simulink model "open_loop_experiments_R2018b"  (R2018b)
settings: Solver=ode45  StartTime=0.0  StopTime=simulation_time  MaxStep=0.01  RelTol=1e-3  EnableMultiTasking=on
values from neighbouring files (symbols this model uses):
  A = zeros(5,5)    [ex1.m]
  B = zeros(5,2)    [ex1.m]
  C = eye(5)    [ex1.m]    (also in exercise2_LQRandObserver.m = Corig)
  D = zeros(5,2)    [ex1.m]
  parameters = sol.getSystemParameters    [exercise1_Linearization.m]    (also in exercise2_LQRandObserver.m = sol1.getSystemParameters)
  path_to_track = ut.genCircularPath(curvature)    [exercise1_Linearization.m]
  Phi = eye(5) + A.*sampling_time*Psi    [ex1.m]
  sampling_time = 0.1    [exercise1_Linearization.m]    (also in exercise2_LQRandObserver.m = 0.01)
  x0 = {x0_experiment_1}    [ex1.m]    (also in exercise1_Linearization.m = x0_experiments{exp_id})
  x0_tild = x0Tild_experiments{exp_id}    [exercise1_Linearization.m]
undefined symbols (not defined in the file or in its folder): Gam
settings Model: Creator=ezequiel  LastModifiedBy=jianh
settings OptimizationCC: LifeSpan=inf
settings DebuggingCC: AllowSymbolicDim=off  SFUnexpectedBacktrackingDiag=warning  SFNoUnconditionalDefaultTransitionDiag=warning  SFExecutionAtInitializationDiag=none
settings ModelReferenceCC: PropagateSignalLabelsOutOfModel=off
settings SFSimCC: SimUseLocalCustomCode=off
settings RTWCC: RTWUseLocalCustomCode=off
settings CodeAppCC: StateflowObjectComments=on
settings GRTTargetCC: TargetLangStandard=C89/C90 (ANSI)
settings ConfigComp: CovMetricSettings=dw  CovHtmlReporting=on  CovSaveCumulativeToWorkspaceVar=on  CovSaveSingleToWorkspaceVar=on  CovExternalEMLEnable=off

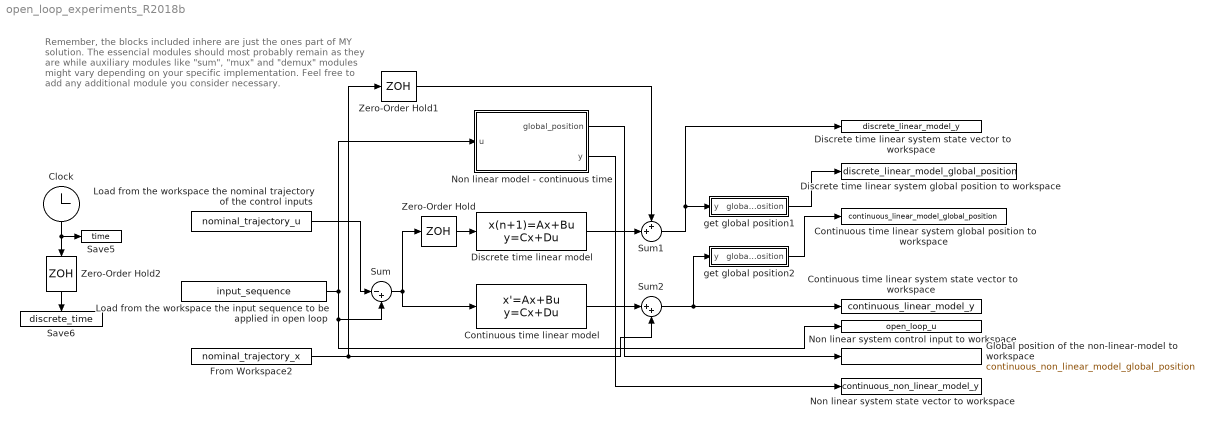
== system open_loop_experiments_R2018b ==
  note: Remember, the blocks included inhere are just the ones part of MY solution. The essencial modules should most probably remain as they are while auxiliary modules like "sum", "mux" and "demux" modules might vary depending on your specific implementation.
      |
      | Feel free to add any additional module you consider necessary.
  " Discrete time linear system state vector to workspace" : ToWorkspace  VariableName=discrete_linear_model_y  SampleTime=-1
  Clock : Clock
  Continuous time linear model : StateSpace  A=A  B=B  C=C  D=D  InitialCondition=x0_tild
  Continuous time linear system global position to workspace : ToWorkspace  VariableName=continuous_linear_model_global_position  SampleTime=-1
  Continuous time linear system state vector to workspace : ToWorkspace  VariableName=continuous_linear_model_y  SampleTime=-1
  Discrete time linear model : DiscreteStateSpace  A=Phi  B=Gam  C=C  D=D  InitialCondition=x0_tild  SampleTime=sampling_time
  Discrete time linear system global position to workspace : ToWorkspace  VariableName=discrete_linear_model_global_position  SampleTime=-1
  From Workspace2 : FromWorkspace  VariableName=nominal_trajectory_x  SampleTime=sampling_time  Interpolate=off  OutputAfterFinalValue=Holding final value
  Global position of the non-linear-model to workspace : ToWorkspace  VariableName=continuous_non_linear_model_global_position  SampleTime=-1
  Load from the workspace the input sequence to be applied in open loop : FromWorkspace  VariableName=input_sequence  SampleTime=sampling_time
  Load from the workspace the nominal trajectory of the control inputs : FromWorkspace  VariableName=nominal_trajectory_u  SampleTime=sampling_time  Interpolate=off  OutputAfterFinalValue=Holding final value
  Non linear model - continuous time : Subsystem
  Non linear system control input to workspace : ToWorkspace  VariableName=open_loop_u  SampleTime=-1
  Non linear system state vector to workspace : ToWorkspace  VariableName=continuous_non_linear_model_y  SampleTime=-1
  Save5 : ToWorkspace  VariableName=time  SampleTime=-1
  Save6 : ToWorkspace  VariableName=discrete_time  SampleTime=-1
  Sum : Sum  Inputs=|-+
  Sum1 : Sum  Inputs=++|
  Sum2 : Sum  Inputs=|++
  Zero-Order Hold : ZeroOrderHold  SampleTime=sampling_time
  Zero-Order Hold1 : ZeroOrderHold  SampleTime=sampling_time
  Zero-Order Hold2 : ZeroOrderHold  SampleTime=sampling_time
  get global position1 : Subsystem
  get global position2 : Subsystem
  wires:
  Clock/1 -> Save5/1, Zero-Order Hold2/1
  Zero-Order Hold2/1 -> Save6/1
  Non linear model - continuous time/1(global_position) -> Global position of the non-linear-model to workspace/1
  Sum/1 -> Continuous time linear model/1, Zero-Order Hold/1
  Zero-Order Hold/1 -> Discrete time linear model/1
  get global position1/1(global_position) -> Discrete time linear system global position to workspace/1
  get global position2/1(global_position) -> Continuous time linear system global position to workspace/1
  Non linear model - continuous time/2(y) -> Non linear system state vector to workspace/1
  Load from the workspace the nominal trajectory of the control inputs/1 -> Sum/1
  Load from the workspace the input sequence to be applied in open loop/1 -> Non linear model - continuous time/1(u), Non linear system control input to workspace/1, Sum/2
  Discrete time linear model/1 -> Sum1/2
  Sum1/1 -> " Discrete time linear system state vector to workspace"/1, get global position1/1(y)
  Continuous time linear model/1 -> Sum2/1
  Sum2/1 -> Continuous time linear system state vector to workspace/1, get global position2/1(y)
  From Workspace2/1 -> Zero-Order Hold1/1, Sum2/2
  Zero-Order Hold1/1 -> Sum1/1

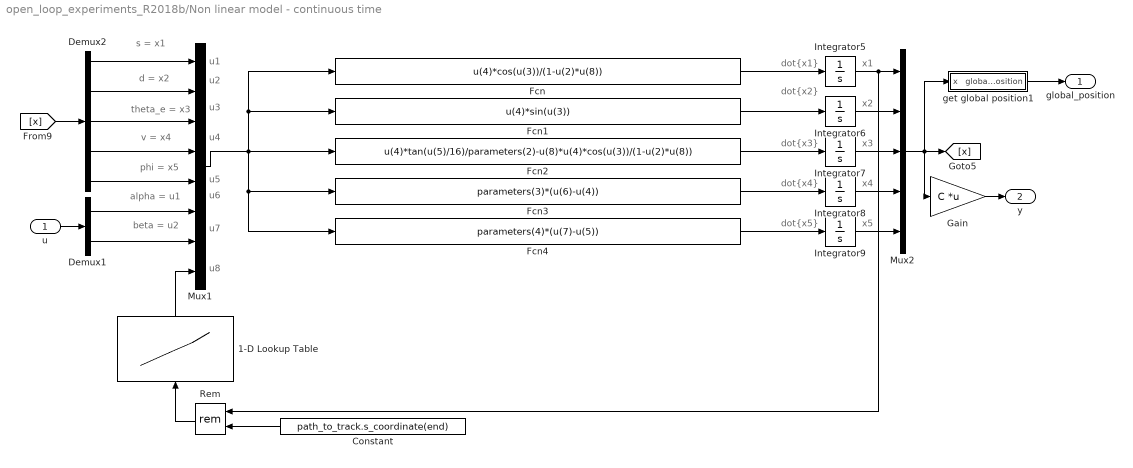
== system open_loop_experiments_R2018b/Non linear model - continuous time ==
  note: s = x1
  note: dot{x1}
  note: d = x2
  note: theta_e = x3
  note: v = x4
  note: phi = x5
  note: alpha = u1
  note: beta = u2
  note: u1
  note: u2
  note: u3
  note: u4
  note: u5
  note: u6
  note: u7
  note: x1
  note: dot{x2}
  note: x2
  note: dot{x3}
  note: x3
  note: dot{x4}
  note: x4
  note: dot{x5}
  note: x5
  note: u8
  u : Inport
  1-D Lookup Table : Lookup_n-D  NumberOfTableDimensions=1  BreakpointsForDimension1=path_to_track.s_coordinate  Table=path_to_track.curvature  InternalRulePriority=Speed  RndMeth=Simplest  InputSameDT=on
  Constant : Constant  Value=path_to_track.s_coordinate(end)
  Demux1 : Demux  Outputs=2
  Demux2 : Demux  Outputs=5
  Fcn : Fcn  Expr=u(4)*cos(u(3))/(1-u(2)*u(8))
  Fcn1 : Fcn  Expr=u(4)*sin(u(3))
  Fcn2 : Fcn  Expr=u(4)*tan(u(5)/16)/parameters(2)-u(8)*u(4)*cos(u(3))/(1-u(2)*u(8))
  Fcn3 : Fcn  Expr=parameters(3)*(u(6)-u(4))
  Fcn4 : Fcn  Expr=parameters(4)*(u(7)-u(5))
  Gain : Gain  Gain=C  Multiplication=Matrix(K*u)
  Integrator5 : Integrator  InitialCondition=x0(1)
  Integrator6 : Integrator  InitialCondition=x0(2)
  Integrator7 : Integrator  InitialCondition=x0(3)
  Integrator8 : Integrator  InitialCondition=x0(4)
  Integrator9 : Integrator  InitialCondition=x0(5)
  Mux1 : Mux  Inputs=8
  Mux2 : Mux  Inputs=5
  Rem : Math  Operator=rem  SaturateOnIntegerOverflow=on
  get global position1 : Subsystem
  global_position : Outport
  y : Outport  Port=2
  wires:
  u/1 -> Demux1/1
  Fcn/1 -> Integrator5/1
  Demux2/1 -> Mux1/1
  Demux2/2 -> Mux1/2
  Demux2/3 -> Mux1/3
  Demux2/4 -> Mux1/4
  Demux2/5 -> Mux1/5
  Demux1/1 -> Mux1/6
  Demux1/2 -> Mux1/7
  Mux1/1 -> Fcn3/1, Fcn4/1, Fcn1/1, Fcn/1, Fcn2/1
  Fcn1/1 -> Integrator6/1
  Integrator6/1 -> Mux2/2
  Fcn2/1 -> Integrator7/1
  Integrator7/1 -> Mux2/3
  Fcn3/1 -> Integrator8/1
  Integrator8/1 -> Mux2/4
  Fcn4/1 -> Integrator9/1
  Integrator9/1 -> Mux2/5
  [x] -> Demux2/1
  1-D Lookup Table/1 -> Mux1/8
  Rem/1 -> 1-D Lookup Table/1
  Constant/1 -> Rem/2
  Integrator5/1 -> Rem/1, Mux2/1
  Mux2/1 -> Gain/1, get global position1/1(x), [x]
  get global position1/1(global_position) -> global_position/1
  Gain/1 -> y/1

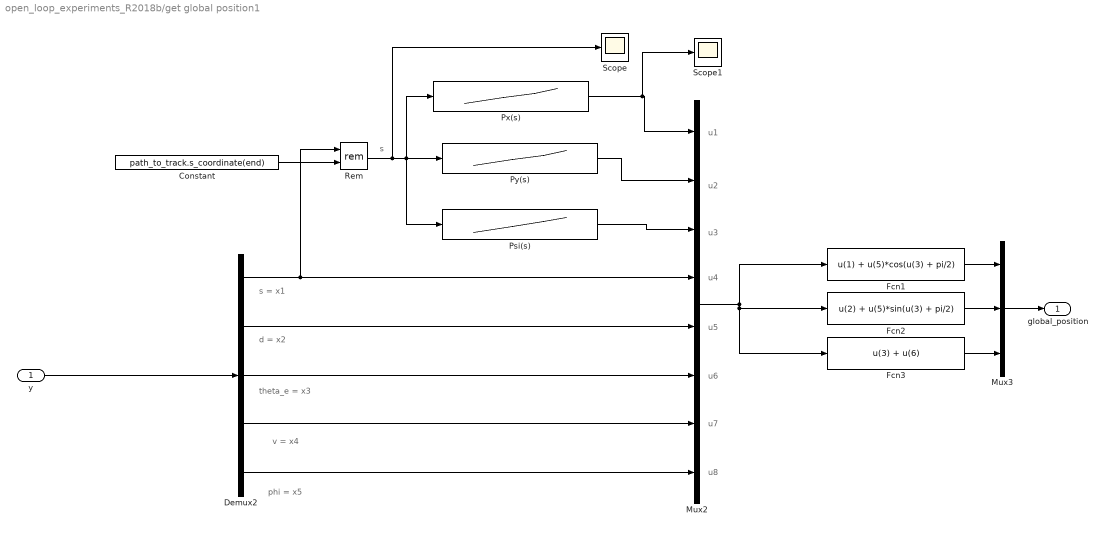
== system open_loop_experiments_R2018b/get global position1 ==
  note: s
  note: s = x1
  note: d = x2
  note: theta_e = x3
  note: v = x4
  note: phi = x5
  note: u1
  note: u2
  note: u3
  note: u4
  note: u5
  note: u6
  note: u7
  note: u8
  y : Inport
  Constant : Constant  Value=path_to_track.s_coordinate(end)
  Demux2 : Demux  Outputs=5
  Fcn1 : Fcn  Expr=u(1) + u(5)*cos(u(3) + pi/2)
  Fcn2 : Fcn  Expr=u(2) + u(5)*sin(u(3) + pi/2)
  Fcn3 : Fcn  Expr=u(3) + u(6)
  Mux2 : Mux  Inputs=8
  Mux3 : Mux  Inputs=3
  Psi(s) : Lookup_n-D  NumberOfTableDimensions=1  BreakpointsForDimension1=path_to_track.s_coordinate  Table=path_to_track.orientation  InternalRulePriority=Speed  RndMeth=Simplest  InputSameDT=on
  Px(s) : Lookup_n-D  NumberOfTableDimensions=1  BreakpointsForDimension1=path_to_track.s_coordinate  Table=path_to_track.coordinates(:,1)  InternalRulePriority=Speed  RndMeth=Simplest  InputSameDT=on
  Py(s) : Lookup_n-D  NumberOfTableDimensions=1  BreakpointsForDimension1=path_to_track.s_coordinate  Table=path_to_track.coordinates(:,2)  InternalRulePriority=Speed  RndMeth=Simplest  InputSameDT=on
  Rem : Math  Operator=rem  SaturateOnIntegerOverflow=on
  Scope : Scope
  Scope1 : Scope
  global_position : Outport
  wires:
  Demux2/1 -> Mux2/4, Rem/1
  Mux3/1 -> global_position/1
  y/1 -> Demux2/1
  Rem/1 -> Scope/1, Psi(s)/1, Px(s)/1, Py(s)/1
  Constant/1 -> Rem/2
  Px(s)/1 -> Scope1/1, Mux2/1
  Py(s)/1 -> Mux2/2
  Psi(s)/1 -> Mux2/3
  Mux2/1 -> Fcn3/1, Fcn2/1, Fcn1/1
  Fcn1/1 -> Mux3/1
  Fcn2/1 -> Mux3/2
  Fcn3/1 -> Mux3/3
  Demux2/2 -> Mux2/5
  Demux2/3 -> Mux2/6
  Demux2/4 -> Mux2/7
  Demux2/5 -> Mux2/8

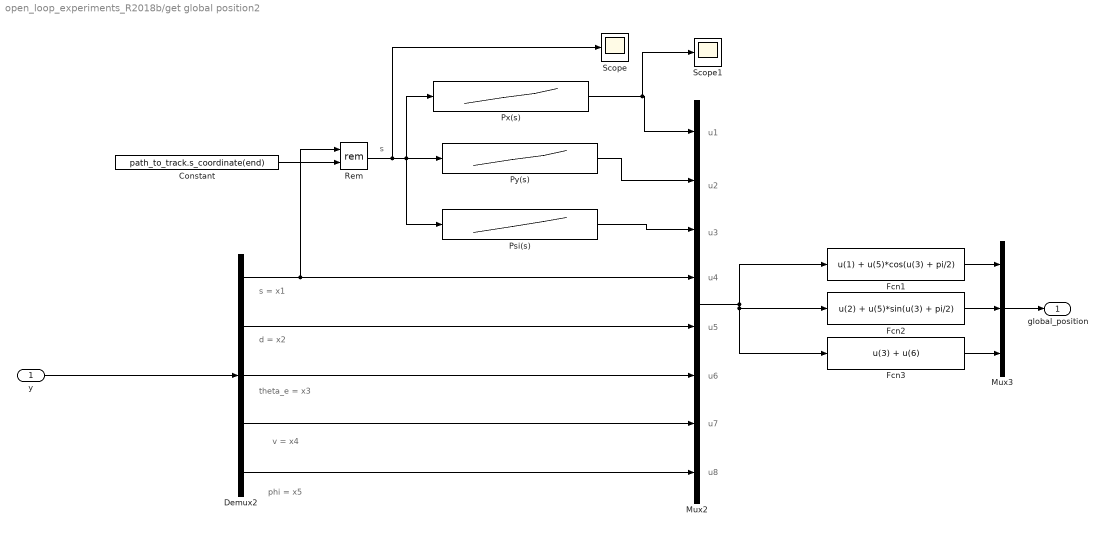
== system open_loop_experiments_R2018b/get global position2 ==
  note: u8
  note: u7
  note: u6
  note: u5
  note: u4
  note: u3
  note: u2
  note: u1
  note: phi = x5
  note: v = x4
  note: theta_e = x3
  note: d = x2
  note: s = x1
  note: s
  y : Inport
  Constant : Constant  Value=path_to_track.s_coordinate(end)
  Demux2 : Demux  Outputs=5
  Fcn1 : Fcn  Expr=u(1) + u(5)*cos(u(3) + pi/2)
  Fcn2 : Fcn  Expr=u(2) + u(5)*sin(u(3) + pi/2)
  Fcn3 : Fcn  Expr=u(3) + u(6)
  Mux2 : Mux  Inputs=8
  Mux3 : Mux  Inputs=3
  Psi(s) : Lookup_n-D  NumberOfTableDimensions=1  BreakpointsForDimension1=path_to_track.s_coordinate  Table=path_to_track.orientation  InternalRulePriority=Speed  RndMeth=Simplest  InputSameDT=on
  Px(s) : Lookup_n-D  NumberOfTableDimensions=1  BreakpointsForDimension1=path_to_track.s_coordinate  Table=path_to_track.coordinates(:,1)  InternalRulePriority=Speed  RndMeth=Simplest  InputSameDT=on
  Py(s) : Lookup_n-D  NumberOfTableDimensions=1  BreakpointsForDimension1=path_to_track.s_coordinate  Table=path_to_track.coordinates(:,2)  InternalRulePriority=Speed  RndMeth=Simplest  InputSameDT=on
  Rem : Math  Operator=rem  SaturateOnIntegerOverflow=on
  Scope : Scope
  Scope1 : Scope
  global_position : Outport
  wires:
  Demux2/5 -> Mux2/8
  Demux2/4 -> Mux2/7
  Demux2/3 -> Mux2/6
  Demux2/2 -> Mux2/5
  Fcn3/1 -> Mux3/3
  Fcn2/1 -> Mux3/2
  Fcn1/1 -> Mux3/1
  Mux2/1 -> Fcn1/1, Fcn2/1, Fcn3/1
  Psi(s)/1 -> Mux2/3
  Py(s)/1 -> Mux2/2
  Px(s)/1 -> Mux2/1, Scope1/1
  Constant/1 -> Rem/2
  Rem/1 -> Py(s)/1, Px(s)/1, Psi(s)/1, Scope/1
  y/1 -> Demux2/1
  Mux3/1 -> global_position/1
  Demux2/1 -> Rem/1, Mux2/4

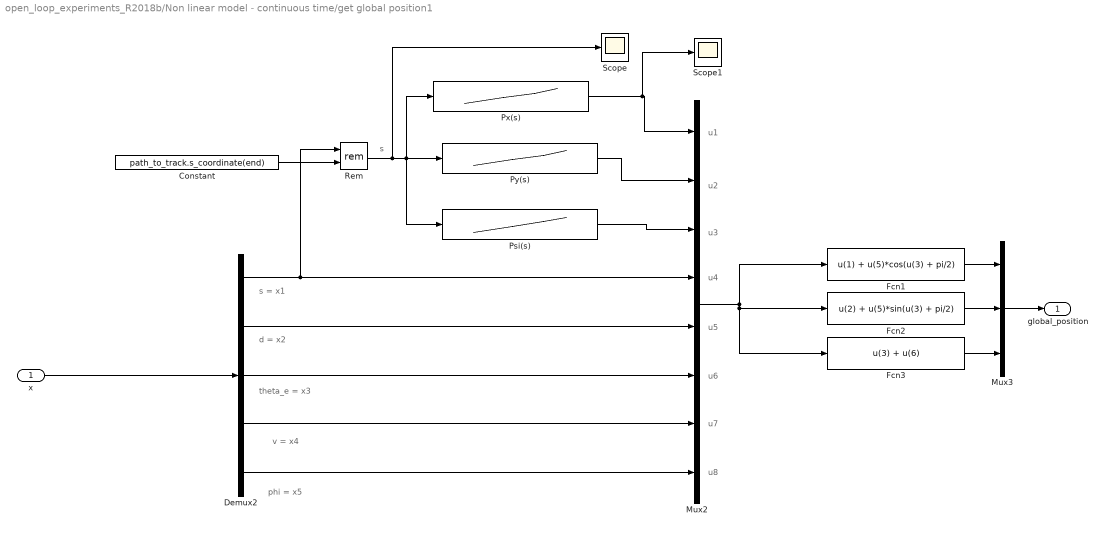
== system open_loop_experiments_R2018b/Non linear model - continuous time/get global position1 ==
  note: s
  note: s = x1
  note: d = x2
  note: theta_e = x3
  note: v = x4
  note: phi = x5
  note: u1
  note: u2
  note: u3
  note: u4
  note: u5
  note: u6
  note: u7
  note: u8
  x : Inport
  Constant : Constant  Value=path_to_track.s_coordinate(end)
  Demux2 : Demux  Outputs=5
  Fcn1 : Fcn  Expr=u(1) + u(5)*cos(u(3) + pi/2)
  Fcn2 : Fcn  Expr=u(2) + u(5)*sin(u(3) + pi/2)
  Fcn3 : Fcn  Expr=u(3) + u(6)
  Mux2 : Mux  Inputs=8
  Mux3 : Mux  Inputs=3
  Psi(s) : Lookup_n-D  NumberOfTableDimensions=1  BreakpointsForDimension1=path_to_track.s_coordinate  Table=path_to_track.orientation  InternalRulePriority=Speed  RndMeth=Simplest  InputSameDT=on
  Px(s) : Lookup_n-D  NumberOfTableDimensions=1  BreakpointsForDimension1=path_to_track.s_coordinate  Table=path_to_track.coordinates(:,1)  InternalRulePriority=Speed  RndMeth=Simplest  InputSameDT=on
  Py(s) : Lookup_n-D  NumberOfTableDimensions=1  BreakpointsForDimension1=path_to_track.s_coordinate  Table=path_to_track.coordinates(:,2)  InternalRulePriority=Speed  RndMeth=Simplest  InputSameDT=on
  Rem : Math  Operator=rem  SaturateOnIntegerOverflow=on
  Scope : Scope
  Scope1 : Scope
  global_position : Outport
  wires:
  Demux2/1 -> Mux2/4, Rem/1
  Mux3/1 -> global_position/1
  x/1 -> Demux2/1
  Rem/1 -> Scope/1, Psi(s)/1, Px(s)/1, Py(s)/1
  Constant/1 -> Rem/2
  Px(s)/1 -> Scope1/1, Mux2/1
  Py(s)/1 -> Mux2/2
  Psi(s)/1 -> Mux2/3
  Mux2/1 -> Fcn3/1, Fcn2/1, Fcn1/1
  Fcn1/1 -> Mux3/1
  Fcn2/1 -> Mux3/2
  Fcn3/1 -> Mux3/3
  Demux2/2 -> Mux2/5
  Demux2/3 -> Mux2/6
  Demux2/4 -> Mux2/7
  Demux2/5 -> Mux2/8
